simulink model "control_esp32_DTS"  (R2026a)
settings: Solver=VariableStepAuto  StopTime=inf
libraries: instrumentseriallib x3
settings Model: Creator=user  LastModifiedBy=jinyu

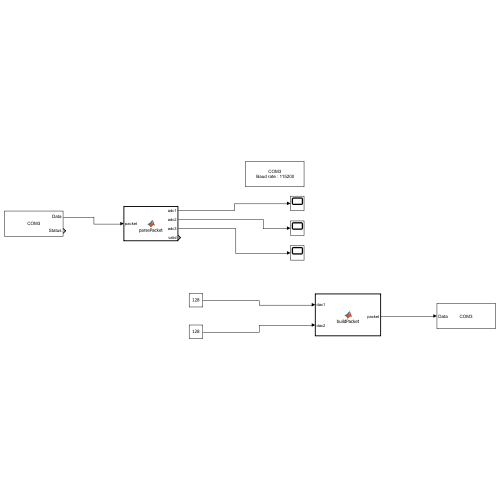
[thumbnail: Simulink's stored preview of the top-level diagram]
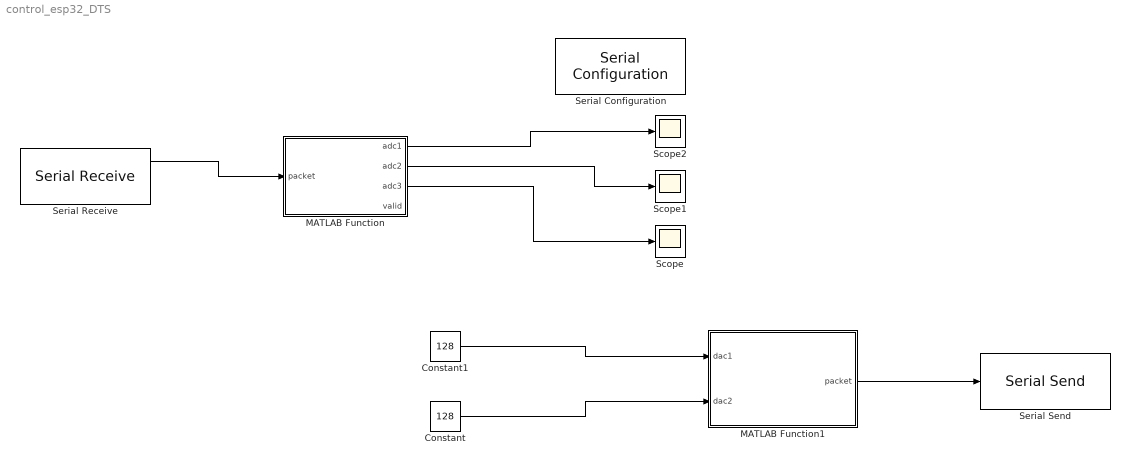
== system control_esp32_DTS ==
  Constant : Constant  Value=128  OutDataTypeStr=uint8
  Constant1 : Constant  Value=128  OutDataTypeStr=uint8
  MATLAB Function : MATLAB Function  TreatAsAtomicUnit=on
  MATLAB Function1 : MATLAB Function  TreatAsAtomicUnit=on
  Scope : Scope
  Scope1 : Scope
  Scope2 : Scope
      settings: DataLoggingVariableName=ScopeData2
  Serial Configuration : instrumentseriallib/Serial Configuration  Priority=-200000  PortSel=COM3  Port=COM3  ComPort=COM3  BaudRate=115200  DataBits=8  Parity=none  StopBits=1  ByteOrder=little-endian  FlowControl=none  Timeout=10  SimulateUsing=Interpreted execution  BlockInModel=on  aMode=1
  Serial Receive : instrumentseriallib/Serial Receive  Priority=1  PortSel=COM3  Port=COM3  ComPort=COM3  DataType=uint8  SaveDataType=uint8  ToggleHeader=on  Header=[0xAA 0x01]  ToggleDataSize=on  DataSize=[9]  ToggleTerminator=off  Terminator=<none>  CustomTerminator=[]  InputFormat=Column major  EnableBlockingMode=off  ActionDataUnavailable=Output last received value  ActionWhenDataUnavailable=Output last received value  CustomValue=0  SampleTime=0.01  SimulateUsing=Interpreted execution  BlockInModel=on  aMode=1  LibraryInUse=instrumentlib
  Serial Send : instrumentseriallib/Serial Send  Priority=1  PortSel=COM3  Port=COM3  ComPort=COM3  Header=[]  Terminator=<none>  CustomTerminator=[]  EnableBlockingMode=off  SimulateUsing=Interpreted execution  BlockInModel=on  aMode=1
  wires:
  MATLAB Function/3(adc3) -> Scope/1
  MATLAB Function/1(adc1) -> Scope2/1
  MATLAB Function/2(adc2) -> Scope1/1
  MATLAB Function1/1(packet) -> Serial Send/1
  Constant1/1 -> MATLAB Function1/1(dac1)
  Constant/1 -> MATLAB Function1/2(dac2)
  Serial Receive/1 -> MATLAB Function/1(packet)

== matlab function control_esp32_DTS/MATLAB Function1 ==
  data: dac1 input; packet output; dac2 input
function packet = buildPacket(dac1, dac2)
    packet = uint8(zeros(5,1));
    packet(1) = hex2dec('BB');
    packet(2) = hex2dec('02');
    packet(3) = uint8(dac1);
    packet(4) = uint8(dac2);
    
    % Calculate checksum
    checksum = uint8(0);
    for i = 1:4
        checksum = bitxor(checksum, packet(i));
    end
    packet(5) = checksum;
end

== matlab function control_esp32_DTS/MATLAB Function ==
  data: packet input; adc1 output; adc2 output; adc3 output; valid output
function [adc1, adc2, adc3, valid] = parsePacket(packet)
    if packet(1) == hex2dec('AA') && packet(2) == hex2dec('01')
        % Verify checksum
        checksum = uint8(0);
        for i = 1:8
            checksum = bitxor(checksum, packet(i));
        end
        if checksum == packet(9)
            % Extract 12-bit ADC values from high and low bytes
            adc1 = double(bitshift(uint16(packet(3)), 8) + uint16(packet(4))) * (3.3 / 4095);
            adc2 = double(bitshift(uint16(packet(5)), 8) + uint16(packet(6))) * (3.3 / 4095);
            adc3 = double(bitshift(uint16(packet(7)), 8) + uint16(packet(8))) * (3.3 / 4095);
            valid = true;
        else
            adc1 = 0; adc2 = 0; adc3 = 0;
            valid = false;
        end
    else
        adc1 = 0; adc2 = 0; adc3 = 0;
        valid = false;
    end
end
